simulink model "Flight_Control_System"  (R2016b)
settings: Solver=ode23t  StartTime=0.0  StopTime=endtime_selfdefine  FixedStep=0.0025  RelTol=1e-3  EnableMultiTasking=on
InitFcn:
  | %load QuadCopterParameters
libraries: vrlib x2, aerolibtransform2 x1, simulink x1
settings Model: Creator=Ehang  LastModifiedBy=GuolongJiang
settings SolverCC: NumberNewtonIterations=2
settings DataIOCC: LimitDataPoints=on  SaveFormat=Array
settings OptimizationCC: ExpressionDepthLimit=2147483647  LifeSpan=inf
settings DebuggingCC: SignalInfNanChecking=error  AlgebraicLoopMsg=error  ArtificialAlgebraicLoopMsg=error  UnderspecifiedInitializationDetection=Classic  MergeDetectMultiDrivingBlocksExec=none  SolverPrmCheckMsg=warning  InheritedTsInSrcMsg=none  FcnCallInpInsideContextMsg=warning  UnconnectedInputMsg=none  UnconnectedOutputMsg=none  UnconnectedLineMsg=none  StateNameClashWarn=warning  SFUnexpectedBacktrackingDiag=warning  SFNoUnconditionalDefaultTransitionDiag=warning  SFExecutionAtInitializationDiag=none
settings HardwareCC: ProdBitPerPointer=32  ProdBitPerSizeT=32  ProdBitPerPtrDiffT=32  ProdLargestAtomicFloat=None  ProdIntDivRoundTo=Undefined  ProdEndianess=Unspecified  ProdWordSize=32  ProdHWDeviceType=32-bit Generic
settings ModelReferenceCC: ModelReferenceNumInstancesAllowed=Single  PropagateSignalLabelsOutOfModel=off
settings GRTTargetCC: TargetLangStandard=C89/C90 (ANSI)  GeneratePreprocessorConditionals=Disable all  CombineOutputUpdateFcns=off  GRTInterface=on
settings ConfigComp: CovMetricSettings=dw  CovHtmlReporting=on  CovSaveCumulativeToWorkspaceVar=on  CovSaveSingleToWorkspaceVar=on  CovExternalEMLEnable=off  CovSFcnEnable=off

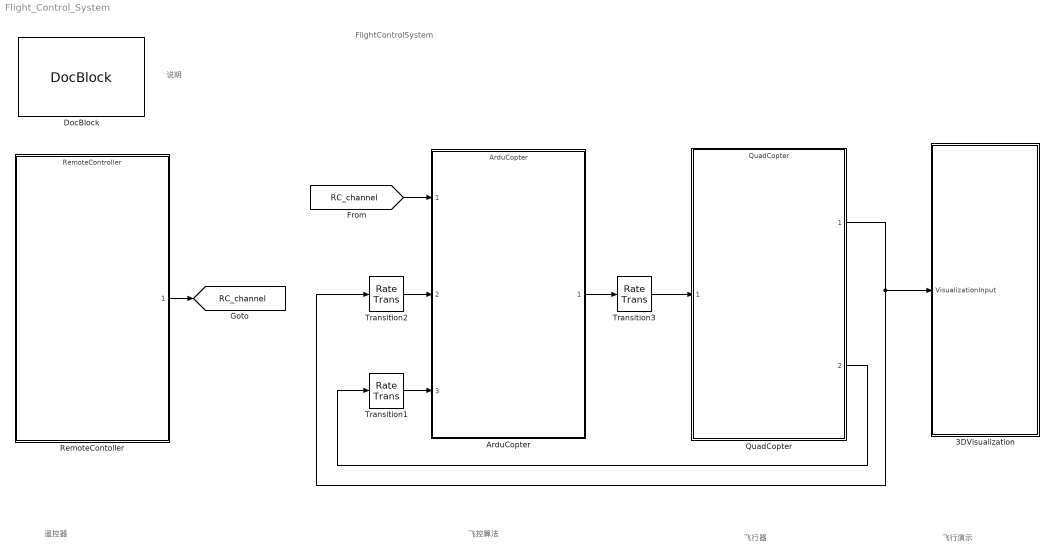
== system Flight_Control_System ==
  note: 说明
  note: 遥控器
  note: FlightControlSystem
  note: 飞控算法
  note: 飞行器
  note: 飞行演示
  3DVisualization : Subsystem  TreatAsAtomicUnit=on
  ArduCopter : ModelReference  ModelNameDialog=ArduCopter  SimulationMode=Normal  ModelReferenceVersion=1.207
  DocBlock : simulink/Model-Wide Utilities/DocBlock  DocumentType=Text  mask(DocBlock){}
      content=|
      | Type your documentation here
      | 主要说明：
      | flight_control_run.m  是运行脚本文件，运行这个文件可以仿真整个模型。
      | Flight_Control_System.slx 是总体模型
      | Remotecontroller.slx 遥控器模型
      | ArduCopter.slx       飞控算法模型
      | QuadCopterSimple.slx 简化版四轴模型
      | QuadCopter.slx       基于物理的四轴模型
      mask Display:
      | % This is a new mask on top of the base mask.
      | % Use "View base mask" link below to see the base mask.
      | image('Ghost2.0.jpg')
  QuadCopter : ModelReference  ModelNameDialog=QuadCopter  SimulationMode=Normal  ModelReferenceVersion=1.202
  RemoteContoller : ModelReference  ModelNameDialog=RemoteController  SimulationMode=Normal  ModelReferenceVersion=1.95
  Transition1 : RateTransition  OutPortSampleTime=0.0025
  Transition2 : RateTransition  OutPortSampleTime=0.0025
  Transition3 : RateTransition  OutPortSampleTime=0
  tag scope: RC_channel=global
  wires:
  [RC_channel] -> ArduCopter/1
  RemoteContoller/1 -> [RC_channel]
  QuadCopter/1 -> Transition2/1, 3DVisualization/1(VisualizationInput)
  ArduCopter/1 -> Transition3/1
  Transition3/1 -> QuadCopter/1
  QuadCopter/2 -> Transition1/1
  Transition2/1 -> ArduCopter/2
  Transition1/1 -> ArduCopter/3

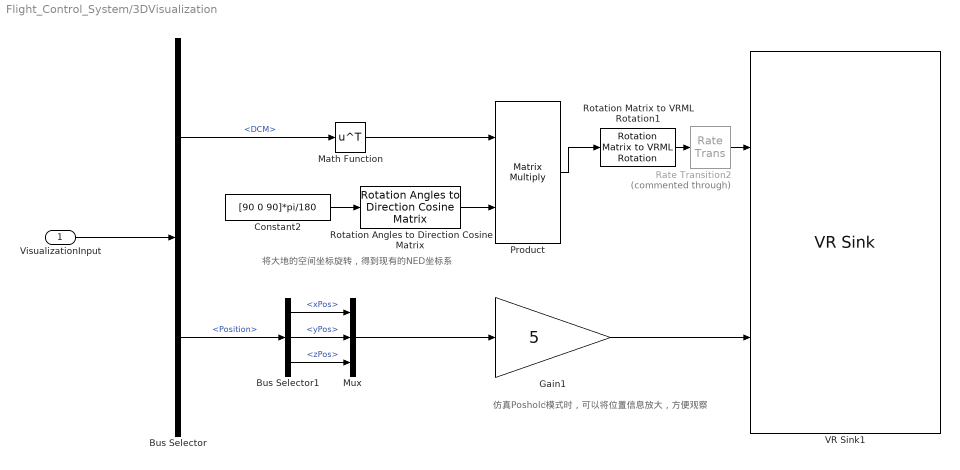
== system Flight_Control_System/3DVisualization ==
  note: 仿真Poshold模式时，可以将位置信息放大，方便观察
  note: 将大地的空间坐标旋转，得到现有的NED坐标系
  VisualizationInput : Inport
  Bus Selector : BusSelector  OutputSignals=NEDState.Attitude.DCM,NEDState.Position
  Bus Selector1 : BusSelector  OutputSignals=xPos,yPos,zPos
  Constant2 : Constant  Value=[90 0 90]*pi/180
  Gain1 : Gain  Gain=5
  Math Function : Math  Operator=transpose  SaturateOnIntegerOverflow=on
  Mux : Mux  Inputs=3
  Product : Product  Multiplication=Matrix(*)
  Rate Transition2 : RateTransition  Commented=through
  Rotation Angles to Direction Cosine Matrix : aerolibtransform2/Rotation Angles to Direction Cosine Matrix  rotationOrder=XYZ
  Rotation Matrix to VRML Rotation1 : vrlib/Utilities/Rotation Matrix to VRML Rotation  maxzero=1e-12
  VR Sink1 : vrlib/VR Sink  InstantiateOnLoad=on  SampleTime=-1  ViewEnable=on  RemoteChange=off  RemoteView=off  FieldsWritten=Drone.rotation.4.1.1.double#Drone.translation.3.1.1.double  WorldFileName=myDrone3.wrl  AutoView=off  VideoDimensions=[]  AllowVariableSize=off
  wires:
  VisualizationInput/1 -> Bus Selector/1
  Rotation Matrix to VRML Rotation1/1 -> Rate Transition2/1
  Rate Transition2/1 -> VR Sink1/1
  Bus Selector/2 -> Bus Selector1/1  "<Position>"
  Mux/1 -> Gain1/1
  Constant2/1 -> Rotation Angles to Direction Cosine Matrix/1
  Rotation Angles to Direction Cosine Matrix/1 -> Product/2
  Math Function/1 -> Product/1
  Product/1 -> Rotation Matrix to VRML Rotation1/1
  Bus Selector/1 -> Math Function/1  "<DCM>"
  Bus Selector1/1 -> Mux/1  "<xPos>"
  Bus Selector1/2 -> Mux/2  "<yPos>"
  Bus Selector1/3 -> Mux/3  "<zPos>"
  Gain1/1 -> VR Sink1/2
